simulink model "FD_5"  (R2015b)
settings: Solver=ode5  SolverMode=SingleTasking  StartTime=0.0  StopTime=10.0  FixedStep=0.01  RelTol=1e-3
values from neighbouring files (symbols this model uses):
  a0 = 3.6102915*d2r    (= 0.0630114736318)    [FlightDyn_Project5.m]
  b = 30    [FlightDyn_Project5.m]
  b0 = 0    [FlightDyn_Project5.m]
  cbar = 11.32    [FlightDyn_Project5.m]
  CDa = 0.00550063*r2d    (= 0.315162883663)    [FlightDyn_Project5.m]
  CDadot = 0    [FlightDyn_Project5.m]
  CDde = -0.000587647*r2d    (= -0.0336696929435)    [FlightDyn_Project5.m]
  CDdf = 0.00136385*r2d    (= 0.0781428488889)    [FlightDyn_Project5.m]
  CDo = 0.01192128    [FlightDyn_Project5.m]
  CDq = 0.00315057*r2d    (= 0.180514364061)    [FlightDyn_Project5.m]
  CLa = 0.0794655*r2d    (= 4.5530377669)    [FlightDyn_Project5.m]
  CLadot = 0    [FlightDyn_Project5.m]
  Clb = -0.00173748*r2d    (= -0.0995502709884)    [FlightDyn_Project5.m]
  Clda = -0.00213984*r2d    (= -0.122603800833)    [FlightDyn_Project5.m]
  CLde = 0.0121988*r2d    (= 0.698939755124)    [FlightDyn_Project5.m]
  CLdf = 0.0144389*r2d    (= 0.827288030811)    [FlightDyn_Project5.m]
  Cldr = 0.000479021*r2d    (= 0.0274458815981)    [FlightDyn_Project5.m]
  CLo = 0.004608463    [FlightDyn_Project5.m]
  Clo = 0    [FlightDyn_Project5.m]
  Clp = -0.00739342*r2d    (= -0.423611762168)    [FlightDyn_Project5.m]
  CLq = 0.0508476*r2d    (= 2.91335287837)    [FlightDyn_Project5.m]
  Clr = 0.0000699792*r2d    (= 0.0040095128137)    [FlightDyn_Project5.m]
  Cma = -0.0041873*r2d    (= -0.239914617555)    [FlightDyn_Project5.m]
  Cmadot = -0.05*r2d    (= -2.86478897565)    [FlightDyn_Project5.m]
  Cmde = -0.0115767*r2d    (= -0.663296050689)    [FlightDyn_Project5.m]
  Cmdf = 0.000580220*r2d    (= 0.0332441571891)    [FlightDyn_Project5.m]
  Cmo = -0.02092347    [FlightDyn_Project5.m]
  Cmq = -0.060661*r2d    (= -3.47561928104)    [FlightDyn_Project5.m]
  Cnb = 0.00320831*r2d    (= 0.18382262237)    [FlightDyn_Project5.m]
  Cnda = -0.000206591*r2d    (= -0.0118367923854)    [FlightDyn_Project5.m]
  Cndr = -0.00144865*r2d    (= -0.0830015309916)    [FlightDyn_Project5.m]
  Cno = 0    [FlightDyn_Project5.m]
  Cnp = -0.000432575*r2d    (= -0.0247847218229)    [FlightDyn_Project5.m]
  Cnr = -0.00886783*r2d    (= -0.508089232439)    [FlightDyn_Project5.m]
  CYb = -0.0219309*r2d    (= -1.25654801092)    [FlightDyn_Project5.m]
  CYda = 0.00049355*r2d    (= 0.0282783319787)    [FlightDyn_Project5.m]
  CYdr = 0.00293048*r2d    (= 0.167904135947)    [FlightDyn_Project5.m]
  CYo = 0    [FlightDyn_Project5.m]
  CYp = 0.00133787*r2d    (= 0.0766543045372)    [FlightDyn_Project5.m]
  CYr = 0.0094053*r2d    (= 0.538883995054)    [FlightDyn_Project5.m]
  daf = 0    [FlightDyn_Project5.m]
  dai = 0    [FlightDyn_Project5.m]
  def = -3.03804303*d2r    (= -0.0530238536908)    [FlightDyn_Project5.m]
  dei = -3.03804303*d2r    (= -0.0530238536908)    [FlightDyn_Project5.m]
  df = 1.5*d2r    (= 0.0261799387799)    [FlightDyn_Project5.m]
  drf = -2*d2r    (= -0.0349065850399)    [FlightDyn_Project5.m]
  dri = 0    [FlightDyn_Project5.m]
  g = 32.17561865    [FlightDyn_Project5.m]
  Iinv = inv(I)    [FlightDyn_Project5.m]
  Ixx = 8890.63    [FlightDyn_Project5.m]
  Ixy = 0    [FlightDyn_Project5.m]
  Ixz = 181.119    [FlightDyn_Project5.m]
  Iyy = 71973.5    [FlightDyn_Project5.m]
  Iyz = 0    [FlightDyn_Project5.m]
  Izz = 77141.1    [FlightDyn_Project5.m]
  mass = 762.8447    [FlightDyn_Project5.m]
  p0 = 0    [FlightDyn_Project5.m]
  phi0 = 0    [FlightDyn_Project5.m]
  psi0 = 0    [FlightDyn_Project5.m]
  q0 = 0    [FlightDyn_Project5.m]
  r0 = 0    [FlightDyn_Project5.m]
  r2d = 180/pi    (= 57.2957795131)    [FlightDyn_Project5.m]
  rho = 0.0014962376    [FlightDyn_Project5.m]
  S = 300    [FlightDyn_Project5.m]
  T = 3146.482666    [FlightDyn_Project5.m]
  theta0 = 3.6102915*d2r    (= 0.0630114736318)    [FlightDyn_Project5.m]
  Vt0 = 626.81863    [FlightDyn_Project5.m]
settings Model: Creator=bsg3163  LastModifiedBy=Ben
settings DataIOCC: SaveFormat=Array
settings OptimizationCC: BlockReduction=off  BooleanDataType=off
settings DebuggingCC: SaveWithParameterizedLinksMsg=none  UnderspecifiedInitializationDetection=Classic  MergeDetectMultiDrivingBlocksExec=none  SignalResolutionControl=TryResolveAllWithWarning
settings HardwareCC: ProdBitPerPointer=32  ProdLargestAtomicFloat=None  ProdIntDivRoundTo=Undefined  ProdEndianess=Unspecified  ProdWordSize=32  ProdHWDeviceType=32-bit Generic  TargetUnknown=on
settings GRTTargetCC: GeneratePreprocessorConditionals=Disable all
settings ConfigComp: CovModelRefEnable=Off  CovSFcnEnable=off

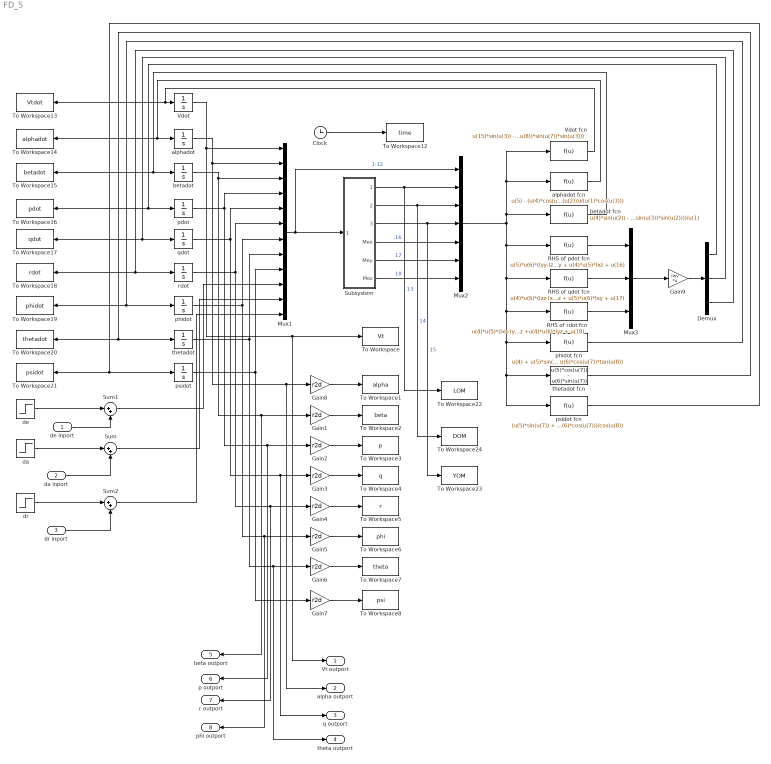
== system FD_5 ==
  de inport : Inport
  da inport : Inport  Port=2
  dr inport : Inport  Port=3
  Clock : Clock
  Demux : Demux  Outputs=3
  Gain{1..8} (8 alike) : Gain  Gain=r2d
  Gain9 : Gain  Gain=Iinv  Multiplication=Matrix(K*u)
  Mux1 : Mux  Inputs=12
  Mux2 : Mux  Inputs=7
  Mux3 : Mux  Inputs=3
  RHS of pdot fcn : Fcn  Expr=u(5)*u(6)*(Iyy-Izz) + ((u(5)^2) - (u(6)^2))*Iyz -u(4)*u(6)*Ixy + u(4)*u(5)*Ixz + u(16)
  RHS of qdot fcn : Fcn  Expr=u(4)*u(6)*(Izz-Ixx) + ((u(6)^2) - (u(4)^2))*Ixz - u(4)*u(5)*Iyz + u(5)*u(6)*Ixy + u(17)
  RHS of rdot fcn : Fcn  Expr=u(4)*u(5)*(Ixx-Iyy)+(u(4)^2- u(5)^2)*Ixy - u(5)*u(6)*Ixz +u(4)*u(6)*Iyz + u(18)
  Subsystem : Subsystem
  Sum : Sum  Inputs=|++
  Sum1 : Sum  Inputs=|++
  Sum2 : Sum  Inputs=|++
  To Workspace : ToWorkspace  VariableName=Vt  SampleTime=-1
  To Workspace1 : ToWorkspace  VariableName=alpha  SampleTime=-1
  To Workspace12 : ToWorkspace  VariableName=time  SampleTime=-1
  To Workspace13 : ToWorkspace  VariableName=Vtdot  SampleTime=-1
  To Workspace14 : ToWorkspace  VariableName=alphadot  SampleTime=-1
  To Workspace15 : ToWorkspace  VariableName=betadot  SampleTime=-1
  To Workspace16 : ToWorkspace  VariableName=pdot  SampleTime=-1
  To Workspace17 : ToWorkspace  VariableName=qdot  SampleTime=-1
  To Workspace18 : ToWorkspace  VariableName=rdot  SampleTime=-1
  To Workspace19 : ToWorkspace  VariableName=phidot  SampleTime=-1
  To Workspace2 : ToWorkspace  VariableName=beta  SampleTime=-1
  To Workspace20 : ToWorkspace  VariableName=thetadot  SampleTime=-1
  To Workspace21 : ToWorkspace  VariableName=psidot  SampleTime=-1
  To Workspace22 : ToWorkspace  VariableName=LOM  SampleTime=-1
  To Workspace23 : ToWorkspace  VariableName=YOM  SampleTime=-1
  To Workspace24 : ToWorkspace  VariableName=DOM  SampleTime=-1
  To Workspace3 : ToWorkspace  VariableName=p  SampleTime=-1
  To Workspace4 : ToWorkspace  VariableName=q  SampleTime=-1
  To Workspace5 : ToWorkspace  VariableName=r  SampleTime=-1
  To Workspace6 : ToWorkspace  VariableName=phi  SampleTime=-1
  To Workspace7 : ToWorkspace  VariableName=theta  SampleTime=-1
  To Workspace8 : ToWorkspace  VariableName=psi  SampleTime=-1
  Vdot : Integrator  InitialCondition=Vt0
  Vdot fcn : Fcn  Expr=u(15)*sin(u(3)) - u(14)*cos(u(3)) + g*((cos(u(8))*cos(u(7))*sin(u(2)) - sin(u(8))*cos(u(2)))*cos(u(3)) + cos(u(8))*sin(u(7))*sin(u(3)))
  alphadot : Integrator  InitialCondition=a0
  alphadot fcn : Fcn  Expr=u(5) - (u(4)*cos(u(2)) + u(6)*sin(u(2)))*tan(u(3)) - u(13)/(u(1)*cos(u(3))) + (g*(cos(u(8))*cos(u(7))*cos(u(2)) + sin(u(8))*sin(u(2))))/(u(1)*cos(u(3)))
  betadot : Integrator  InitialCondition=b0
  betadot fcn : Fcn  Expr=u(4)*sin(u(2)) - u(6)*cos(u(2)) + (u(15)*cos(u(3)) + u(14)*sin(u(3)))/u(1) + (g*(cos(u(8))*sin(u(7))*cos(u(3)) + sin(u(8))*sin(u(3))*cos(u(2)) - cos(u(8))*cos(u(7))*sin(u(3))*sin(u(2))))/u(1)
  da : Step  Before=dai  After=daf  SampleTime=0
  de : Step  Before=dei  After=def  SampleTime=0
  dr : Step  Before=dri  After=drf  SampleTime=0
  pdot : Integrator  InitialCondition=p0
  phidot : Integrator  InitialCondition=phi0
  phidot fcn : Fcn  Expr=u(4) + u(5)*sin(u(7))*tan(u(8)) + u(6)*cos(u(7))*tan(u(8))
  psidot : Integrator  InitialCondition=psi0
  psidot fcn : Fcn  Expr=(u(5)*sin(u(7)) + u(6)*cos(u(7)))/cos(u(8))
  qdot : Integrator  InitialCondition=q0
  rdot : Integrator  InitialCondition=r0
  thetadot : Integrator  InitialCondition=theta0
  thetadot fcn : Fcn  Expr=u(5)*cos(u(7)) - u(6)*sin(u(7))
  Vt outport : Outport
  alpha outport : Outport  Port=2
  q outport : Outport  Port=3
  theta outport : Outport  Port=4
  beta outport : Outport  Port=5
  p outport : Outport  Port=6
  r outport : Outport  Port=7
  phi outport : Outport  Port=8
  wires:
  Mux1/1 -> Subsystem/1(Signals), Mux2/1  "1-12"
  Subsystem/1(LOM) -> To Workspace22/1, Mux2/2  "13"
  Subsystem/2(DOM) -> To Workspace24/1, Mux2/3  "14"
  Subsystem/3(YOM) -> To Workspace23/1, Mux2/4  "15"
  Subsystem/4(Mex) -> Mux2/5  "16"
  Subsystem/5(Mey) -> Mux2/6  "17"
  Subsystem/6(Mez) -> Mux2/7  "18"
  Vdot/1 -> Vt outport/1, To Workspace/1, Mux1/1
  psidot/1 -> Gain7/1, Mux1/9
  Gain8/1 -> To Workspace1/1
  Gain1/1 -> To Workspace2/1
  Gain2/1 -> To Workspace3/1
  Gain3/1 -> To Workspace4/1
  Gain4/1 -> To Workspace5/1
  Gain5/1 -> To Workspace6/1
  Gain6/1 -> To Workspace7/1
  Gain7/1 -> To Workspace8/1
  thetadot/1 -> theta outport/1, Gain6/1, Mux1/8
  phidot/1 -> Gain5/1, phi outport/1, Mux1/7
  rdot/1 -> Gain4/1, r outport/1, Mux1/6
  qdot/1 -> q outport/1, Gain3/1, Mux1/5
  pdot/1 -> Mux1/4, p outport/1, Gain2/1
  betadot/1 -> beta outport/1, Gain1/1, Mux1/3
  alphadot/1 -> alpha outport/1, Gain8/1, Mux1/2
  Mux2/1 -> RHS of rdot fcn/1, psidot fcn/1, thetadot fcn/1, phidot fcn/1, RHS of qdot fcn/1, RHS of pdot fcn/1, alphadot fcn/1, Vdot fcn/1, betadot fcn/1
  RHS of pdot fcn/1 -> Mux3/1
  RHS of qdot fcn/1 -> Mux3/2
  RHS of rdot fcn/1 -> Mux3/3
  Mux3/1 -> Gain9/1
  Gain9/1 -> Demux/1
  Demux/1 -> To Workspace16/1, pdot/1
  Demux/2 -> To Workspace17/1, qdot/1
  Demux/3 -> To Workspace18/1, rdot/1
  Vdot fcn/1 -> To Workspace13/1, Vdot/1
  alphadot fcn/1 -> alphadot/1, To Workspace14/1
  betadot fcn/1 -> betadot/1, To Workspace15/1
  phidot fcn/1 -> phidot/1, To Workspace19/1
  thetadot fcn/1 -> To Workspace20/1, thetadot/1
  psidot fcn/1 -> psidot/1, To Workspace21/1
  Clock/1 -> To Workspace12/1
  Sum/1 -> Mux1/11
  da/1 -> Sum/1
  dr/1 -> Sum2/1
  Sum2/1 -> Mux1/12
  de/1 -> Sum1/1
  Sum1/1 -> Mux1/10
  de inport/1 -> Sum1/2
  da inport/1 -> Sum/2
  dr inport/1 -> Sum2/2

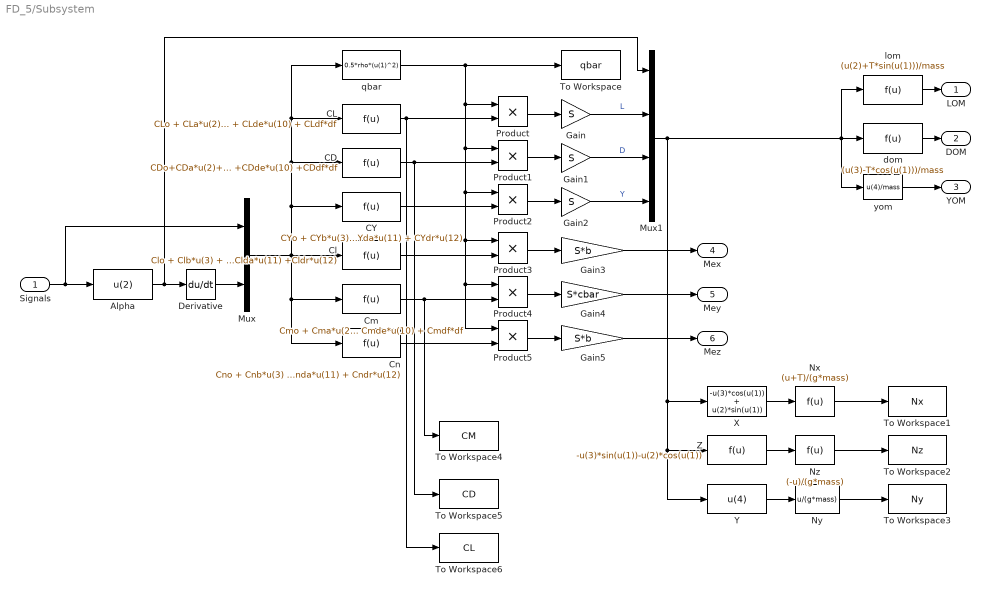
== system FD_5/Subsystem ==
  Signals : Inport
  Alpha : Fcn  Expr=u(2)
  CD : Fcn  Expr=CDo+CDa*u(2)+(cbar/(2*u(1)))*(CDq*u(5)+CDadot*u(13)) +CDde*u(10) +CDdf*df
  CL : Fcn  Expr=CLo + CLa*u(2) + (cbar/(2*u(1)))*(CLq*u(5) + CLadot*u(13)) + CLde*u(10) + CLdf*df
  CY : Fcn  Expr=CYo + CYb*u(3) + (b/(2*u(1)))*(CYp*u(4)+CYr*u(6))+ CYda*u(11) + CYdr*u(12)
  Cl : Fcn  Expr=Clo + Clb*u(3) + (b/(2*u(1)))*(Clp*u(4) + Clr*u(6)) +Clda*u(11) +Cldr*u(12)
  Cm : Fcn  Expr=Cmo + Cma*u(2) + (cbar/(2*u(1)))*(Cmq*u(5) + Cmadot*u(13)) + Cmde*u(10) + Cmdf*df
  Cn : Fcn  Expr=Cno + Cnb*u(3) + (b/(2*u(1)))*(Cnp*u(4) + Cnr*u(6)) + Cnda*u(11) + Cndr*u(12)
  Derivative : Derivative
  Gain : Gain  Gain=S
  Gain1 : Gain  Gain=S
  Gain2 : Gain  Gain=S
  Gain3 : Gain  Gain=S*b
  Gain4 : Gain  Gain=S*cbar
  Gain5 : Gain  Gain=S*b
  Mux : Mux  Inputs=2
  Mux1 : Mux
  Nx : Fcn  Expr=(u+T)/(g*mass)
  Ny : Fcn  Expr=u/(g*mass)
  Nz : Fcn  Expr=(-u)/(g*mass)
  Product{,1..5} (6 alike) : Product
  To Workspace : ToWorkspace  VariableName=qbar  SampleTime=-1
  To Workspace1 : ToWorkspace  VariableName=Nx  SampleTime=-1
  To Workspace2 : ToWorkspace  VariableName=Nz  SampleTime=-1
  To Workspace3 : ToWorkspace  VariableName=Ny  SampleTime=-1
  To Workspace4 : ToWorkspace  VariableName=CM  SampleTime=-1
  To Workspace5 : ToWorkspace  VariableName=CD  SampleTime=-1
  To Workspace6 : ToWorkspace  VariableName=CL  SampleTime=-1
  X : Fcn  Expr=-u(3)*cos(u(1)) + u(2)*sin(u(1))
  Y : Fcn  Expr=u(4)
  Z : Fcn  Expr=-u(3)*sin(u(1))-u(2)*cos(u(1))
  dom : Fcn  Expr=(u(3)-T*cos(u(1)))/mass
  lom : Fcn  Expr=(u(2)+T*sin(u(1)))/mass
  qbar : Fcn  Expr=0.5*rho*(u(1)^2)
  yom : Fcn  Expr=u(4)/mass
  LOM : Outport
  DOM : Outport  Port=2
  YOM : Outport  Port=3
  Mex : Outport  Port=4
  Mey : Outport  Port=5
  Mez : Outport  Port=6
  wires:
  Product1/1 -> Gain1/1
  Product3/1 -> Gain3/1
  CY/1 -> Product2/2
  Derivative/1 -> Mux/2
  Product4/1 -> Gain4/1
  CD/1 -> To Workspace5/1, Product1/2
  Mux/1 -> qbar/1, CL/1, CD/1, CY/1, Cm/1, Cn/1, Cl/1
  Gain1/1 -> Mux1/3  "D"
  Y/1 -> Ny/1
  Nx/1 -> To Workspace1/1
  Mux1/1 -> X/1, Z/1, Y/1, lom/1, yom/1, dom/1
  Z/1 -> Nz/1
  Cn/1 -> Product5/2
  CL/1 -> To Workspace6/1, Product/2
  qbar/1 -> To Workspace/1, Product1/1, Product2/1, Product3/1, Product4/1, Product5/1, Product/1
  Product5/1 -> Gain5/1
  Gain/1 -> Mux1/2  "L"
  Product2/1 -> Gain2/1
  Cl/1 -> Product3/2
  Cm/1 -> To Workspace4/1, Product4/2
  Product/1 -> Gain/1
  Gain2/1 -> Mux1/4  "Y"
  X/1 -> Nx/1
  Nz/1 -> To Workspace2/1
  Ny/1 -> To Workspace3/1
  Signals/1 -> Mux/1, Alpha/1
  Alpha/1 -> Mux1/1, Derivative/1
  lom/1 -> LOM/1
  yom/1 -> YOM/1
  dom/1 -> DOM/1
  Gain4/1 -> Mey/1
  Gain3/1 -> Mex/1
  Gain5/1 -> Mez/1
